simulink model "ControlPendulo2GDL_PL"  (R2019b)
settings: Solver=ode4  StartTime=0.0  StopTime=ts  FixedStep=0.01  RelTol=1e-3
values from neighbouring files (symbols this model uses):
  C = [1 0 0 0]    [PenduloDatos.m]
  K = place(Al,Bl,[Pd1 Pd2 Pd3 Pd4])    [PenduloDatos.m]
  K0 = inv(C*(inv(-Al+Bl*K))*Bl)    [PenduloDatos.m]
  K0D = inv(CD*inv(eye(4)-AD+BD*KD)*BD)    [PenduloDatos.m]
  KD = place(AD,BD,exp([Pd1 Pd2 Pd3 Pd4]*tm))    [PenduloDatos.m]
  L = place(Al',C',[5*Pd1 5*Pd2 5*Pd3 5*Pd4])'    [PenduloDatos.m]
  l1 = c1    (= 0.3)    [PenduloDatos.m]
  l2 = c2    (= 0.2)    [PenduloDatos.m]
  LD = place(AD',CD',exp([5*Pd1 5*Pd2 5*Pd3 5*Pd4]*tm))'    [PenduloDatos.m]
  Ref = 0.2    [PenduloDatos.m]
  tm = 0.01    [PenduloDatos.m]
  XI = [0;0;0;0]    [PenduloDatos.m]
undefined symbols (not defined in the file or in its folder): AD, Al, BD, Bl, CD
libraries: simulink x6
settings Model: Creator=ARQ SEVILLA R  LastModifiedBy=ARQ SEVILLA R

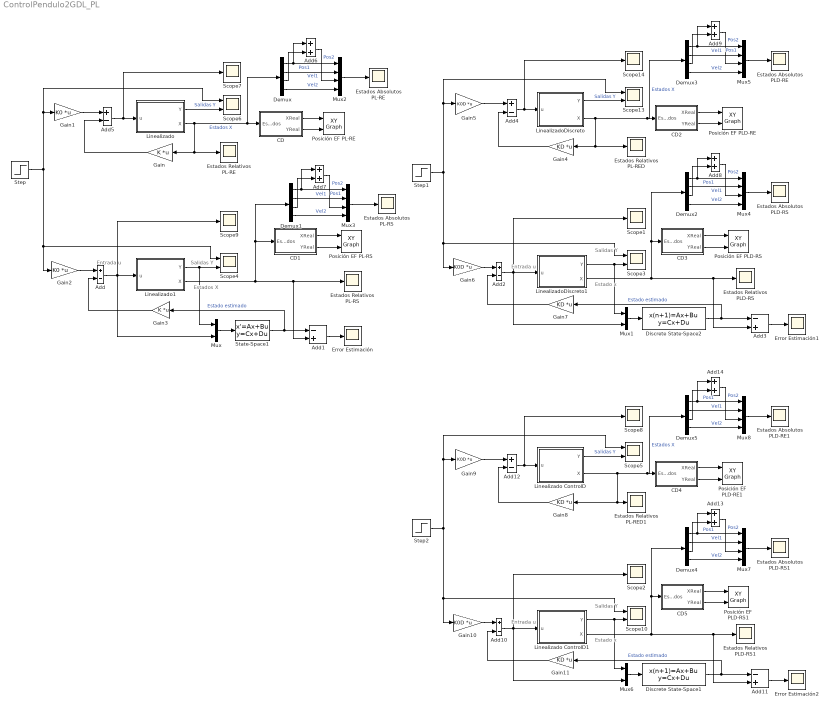
== system ControlPendulo2GDL_PL ==
  note: Estados X
  note: Salidas Y
  note: Entrada u
  note: Salidas Y
  note: Entrada u
  note: Estado x
  note: Entrada u
  note: Estado x
  note: Salidas Y
  Add{,2,4..5,10,12} (6 alike) : Sum  Inputs=+-
  Add1 : Sum  Inputs=-+
  Add11 : Sum  Inputs=-+
  Add{6..9,13..14} (6 alike) : Sum
  Add3 : Sum  Inputs=-+
  CD : Subsystem  TreatAsAtomicUnit=on
  CD1 : Subsystem  TreatAsAtomicUnit=on
  CD2 : Subsystem  TreatAsAtomicUnit=on
  CD3 : Subsystem  TreatAsAtomicUnit=on
  CD4 : Subsystem  TreatAsAtomicUnit=on
  CD5 : Subsystem  TreatAsAtomicUnit=on
  Demux{,1..5} (6 alike) : Demux
  Discrete State-Space1 : DiscreteStateSpace  A=AD-LD*CD  B=[LD BD]  C=eye(4)  D=zeros(4,2)  InitialCondition=XI  SampleTime=tm
  Discrete State-Space2 : DiscreteStateSpace  A=AD-LD*CD  B=[LD BD]  C=eye(4)  D=zeros(4,2)  InitialCondition=XI  SampleTime=tm
  Error Estimación : Scope
  Error Estimación1 : Scope
  Error Estimación2 : Scope
  Estados Absolutos PL-RE : Scope
  Estados Absolutos PL-RS : Scope
  Estados Absolutos PLD-RE : Scope
  Estados Absolutos PLD-RE1 : Scope
  Estados Absolutos PLD-RS : Scope
  Estados Absolutos PLD-RS1 : Scope
  Estados Relativos PL-RE : Scope
  Estados Relativos PL-RED : Scope
  Estados Relativos PL-RED1 : Scope
  Estados Relativos PL-RS : Scope
  Estados Relativos PLD-RS : Scope
  Estados Relativos PLD-RS1 : Scope
  Gain : Gain  Gain=K  Multiplication=Matrix(K*u)
  Gain1 : Gain  Gain=K0  Multiplication=Matrix(K*u)
  Gain{5..6,9..10} (4 alike) : Gain  Gain=K0D  Multiplication=Matrix(K*u)
  Gain{4,7..8,11} (4 alike) : Gain  Gain=KD  Multiplication=Matrix(K*u)
  Gain2 : Gain  Gain=K0  Multiplication=Matrix(K*u)
  Gain3 : Gain  Gain=K  Multiplication=Matrix(K*u)
  Linealizado : Subsystem
  Linealizado ControlD : Subsystem
  Linealizado ControlD1 : Subsystem
  Linealizado1 : Subsystem
  LinealizadoDiscreto : Subsystem
  LinealizadoDiscreto1 : Subsystem
  Mux : Mux  Inputs=2
  Mux1 : Mux  Inputs=2
  Mux{2..5,7..8} (6 alike) : Mux
  Mux6 : Mux  Inputs=2
  Posición EF PL-RE : simulink/Sinks/XY Graph  xmin=-l2-l1  xmax=l2+l1  ymin=-l2-l1  ymax=l2+l1  st=-1
  Posición EF PL-RS : simulink/Sinks/XY Graph  xmin=-l2-l1  xmax=l2+l1  ymin=-l2-l1  ymax=l2+l1  st=-1
  Posición EF PLD-RE : simulink/Sinks/XY Graph  xmin=-l2-l1  xmax=l2+l1  ymin=-l2-l1  ymax=l2+l1  st=-1
  Posición EF PLD-RE1 : simulink/Sinks/XY Graph  xmin=-l2-l1  xmax=l2+l1  ymin=-l2-l1  ymax=l2+l1  st=-1
  Posición EF PLD-RS : simulink/Sinks/XY Graph  xmin=-l2-l1  xmax=l2+l1  ymin=-l2-l1  ymax=l2+l1  st=-1
  Posición EF PLD-RS1 : simulink/Sinks/XY Graph  xmin=-l2-l1  xmax=l2+l1  ymin=-l2-l1  ymax=l2+l1  st=-1
  Scope{1..2,7..9,14} (6 alike) : Scope
  Scope{3..6,10,13} (6 alike) : Scope  NumInputPorts=2
  State-Space1 : StateSpace  A=Al-L*C  B=[L,Bl]  C=eye(4)  D=zeros(4,2)  InitialCondition=XI
  Step : Step  Time=0  After=Ref  SampleTime=0
  Step1 : Step  Time=0  After=Ref  SampleTime=tm
  Step2 : Step  Time=0  After=Ref  SampleTime=tm
  wires:
  Linealizado/2(X) -> Demux/1, CD/1(Estados), Estados Relativos PL-RE/1, Gain/1  "Estados X"
  Add5/1 -> Scope7/1, Linealizado/1(u)
  Gain1/1 -> Add5/1
  Linealizado1/2(X) -> CD1/1(Estados), Demux1/1, Estados Relativos PL-RS/1, Add1/2
  Add/1 -> Scope9/1, Linealizado1/1(u), Mux/2
  Gain2/1 -> Add/1
  Linealizado1/1(Y) -> Mux/1, Scope4/2
  Mux/1 -> State-Space1/1
  Add1/1 -> Error Estimación/1
  Gain3/1 -> Add/2
  State-Space1/1 -> Add1/1, Gain3/1  "Estado estimado"
  CD/1(XReal) -> Posición EF PL-RE/1
  CD/2(YReal) -> Posición EF PL-RE/2
  Step/1 -> Gain2/1, Scope4/1, Scope6/1, Gain1/1
  Linealizado/1(Y) -> Scope6/2  "Salidas Y"
  Gain/1 -> Add5/2
  CD1/2(YReal) -> Posición EF PL-RS/2
  CD1/1(XReal) -> Posición EF PL-RS/1
  LinealizadoDiscreto1/1(Y) -> Mux1/1, Scope3/2
  Gain7/1 -> Add2/2
  LinealizadoDiscreto/1(Y) -> Scope13/2  "Salidas Y"
  Gain6/1 -> Add2/1
  Add2/1 -> Scope1/1, LinealizadoDiscreto1/1(u), Mux1/2
  Add3/1 -> Error Estimación1/1
  Mux1/1 -> Discrete State-Space2/1
  Discrete State-Space2/1 -> Add3/1, Gain7/1  "Estado estimado"
  Gain4/1 -> Add4/2
  Step1/1 -> Scope13/1, Gain5/1, Gain6/1, Scope3/1
  Add4/1 -> LinealizadoDiscreto/1(u), Scope14/1
  Gain5/1 -> Add4/1
  CD2/2(YReal) -> Posición EF PLD-RE/2
  CD2/1(XReal) -> Posición EF PLD-RE/1
  CD3/1(XReal) -> Posición EF PLD-RS/1
  CD3/2(YReal) -> Posición EF PLD-RS/2
  Demux/3 -> Add6/2
  Demux/1 -> Add6/1, Mux2/1  "Pos1"
  Mux2/1 -> Estados Absolutos PL-RE/1
  Demux/2 -> Mux2/2  "Vel1"
  Add6/1 -> Mux2/3  "Pos2"
  Demux/4 -> Mux2/4  "Vel2"
  Demux1/4 -> Mux3/4  "Vel2"
  Add7/1 -> Mux3/3  "Pos2"
  Demux1/2 -> Mux3/2  "Vel1"
  Mux3/1 -> Estados Absolutos PL-RS/1
  Demux1/1 -> Mux3/1, Add7/1  "Pos1"
  Demux1/3 -> Add7/2
  Demux2/3 -> Add8/2
  Demux2/1 -> Add8/1, Mux4/1  "Pos1"
  Mux4/1 -> Estados Absolutos PLD-RS/1
  Demux2/2 -> Mux4/2  "Vel1"
  Add8/1 -> Mux4/3  "Pos2"
  LinealizadoDiscreto1/2(X) -> Estados Relativos PLD-RS/1, Add3/2, Demux2/1, CD3/1(Estados)
  Demux2/4 -> Mux4/4  "Vel2"
  Demux3/4 -> Mux5/4  "Vel2"
  LinealizadoDiscreto/2(X) -> Demux3/1, CD2/1(Estados), Estados Relativos PL-RED/1, Gain4/1  "Estados X"
  Add9/1 -> Mux5/3  "Pos2"
  Demux3/2 -> Mux5/2  "Vel1"
  Mux5/1 -> Estados Absolutos PLD-RE/1
  Demux3/1 -> Mux5/1, Add9/1  "Pos1"
  Demux3/3 -> Add9/2
  Add12/1 -> Linealizado ControlD/1(u), Scope8/1
  Demux4/2 -> Mux7/2  "Vel1"
  Demux4/3 -> Add13/2
  Demux4/1 -> Add13/1, Mux7/1  "Pos1"
  Mux6/1 -> Discrete State-Space1/1
  Linealizado ControlD/1(Y) -> Scope5/2  "Salidas Y"
  Add11/1 -> Error Estimación2/1
  Step2/1 -> Scope5/1, Gain9/1, Gain10/1, Scope10/1
  Add10/1 -> Linealizado ControlD1/1(u), Scope2/1, Mux6/2
  Gain10/1 -> Add10/1
  Linealizado ControlD1/1(Y) -> Mux6/1, Scope10/2
  Demux5/3 -> Add14/2
  Gain9/1 -> Add12/1
  Mux8/1 -> Estados Absolutos PLD-RE1/1
  Linealizado ControlD/2(X) -> Demux5/1, CD4/1(Estados), Gain8/1, Estados Relativos PL-RED1/1  "Estados X"
  Demux5/2 -> Mux8/2  "Vel1"
  Mux7/1 -> Estados Absolutos PLD-RS1/1
  Demux5/1 -> Mux8/1, Add14/1  "Pos1"
  CD4/1(XReal) -> Posición EF PLD-RE1/1
  CD5/2(YReal) -> Posición EF PLD-RS1/2
  Demux4/4 -> Mux7/4  "Vel2"
  CD5/1(XReal) -> Posición EF PLD-RS1/1
  CD4/2(YReal) -> Posición EF PLD-RE1/2
  Gain8/1 -> Add12/2
  Gain11/1 -> Add10/2
  Demux5/4 -> Mux8/4  "Vel2"
  Add14/1 -> Mux8/3  "Pos2"
  Linealizado ControlD1/2(X) -> Estados Relativos PLD-RS1/1, Add11/2, Demux4/1, CD5/1(Estados)
  Discrete State-Space1/1 -> Add11/1, Gain11/1  "Estado estimado"
  Add13/1 -> Mux7/3  "Pos2"

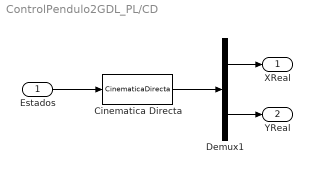
== system ControlPendulo2GDL_PL/CD ==
  Estados : Inport
  Cinematica Directa : MATLABFcn  MATLABFcn=CinematicaDirecta  OutputDimensions=2
  Demux1 : Demux  Outputs=2
  XReal : Outport  VectorParamsAs1DForOutWhenUnconnected=off
  YReal : Outport  Port=2  VectorParamsAs1DForOutWhenUnconnected=off
  wires:
  Cinematica Directa/1 -> Demux1/1
  Demux1/1 -> XReal/1
  Demux1/2 -> YReal/1
  Estados/1 -> Cinematica Directa/1

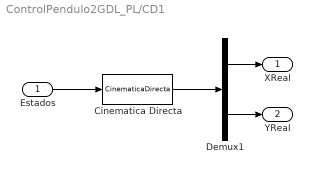
== system ControlPendulo2GDL_PL/CD1 ==
  Estados : Inport
  Cinematica Directa : MATLABFcn  MATLABFcn=CinematicaDirecta  OutputDimensions=2
  Demux1 : Demux  Outputs=2
  XReal : Outport  VectorParamsAs1DForOutWhenUnconnected=off
  YReal : Outport  Port=2  VectorParamsAs1DForOutWhenUnconnected=off
  wires:
  Estados/1 -> Cinematica Directa/1
  Demux1/2 -> YReal/1
  Demux1/1 -> XReal/1
  Cinematica Directa/1 -> Demux1/1

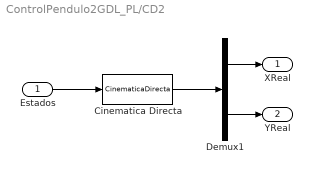
== system ControlPendulo2GDL_PL/CD2 ==
  Estados : Inport
  Cinematica Directa : MATLABFcn  MATLABFcn=CinematicaDirecta  OutputDimensions=2
  Demux1 : Demux  Outputs=2
  XReal : Outport  VectorParamsAs1DForOutWhenUnconnected=off
  YReal : Outport  Port=2  VectorParamsAs1DForOutWhenUnconnected=off
  wires:
  Estados/1 -> Cinematica Directa/1
  Demux1/2 -> YReal/1
  Demux1/1 -> XReal/1
  Cinematica Directa/1 -> Demux1/1

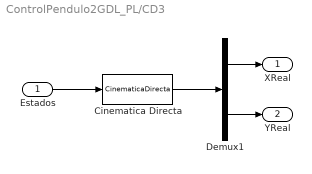
== system ControlPendulo2GDL_PL/CD3 ==
  Estados : Inport
  Cinematica Directa : MATLABFcn  MATLABFcn=CinematicaDirecta  OutputDimensions=2
  Demux1 : Demux  Outputs=2
  XReal : Outport  VectorParamsAs1DForOutWhenUnconnected=off
  YReal : Outport  Port=2  VectorParamsAs1DForOutWhenUnconnected=off
  wires:
  Cinematica Directa/1 -> Demux1/1
  Demux1/1 -> XReal/1
  Demux1/2 -> YReal/1
  Estados/1 -> Cinematica Directa/1

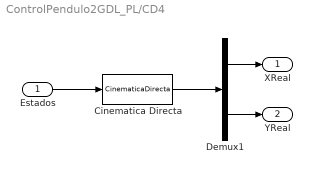
== system ControlPendulo2GDL_PL/CD4 ==
  Estados : Inport
  Cinematica Directa : MATLABFcn  MATLABFcn=CinematicaDirecta  OutputDimensions=2
  Demux1 : Demux  Outputs=2
  XReal : Outport  VectorParamsAs1DForOutWhenUnconnected=off
  YReal : Outport  Port=2  VectorParamsAs1DForOutWhenUnconnected=off
  wires:
  Estados/1 -> Cinematica Directa/1
  Demux1/2 -> YReal/1
  Demux1/1 -> XReal/1
  Cinematica Directa/1 -> Demux1/1

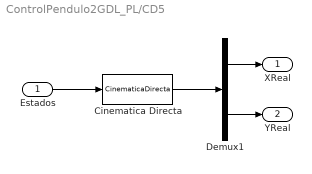
== system ControlPendulo2GDL_PL/CD5 ==
  Estados : Inport
  Cinematica Directa : MATLABFcn  MATLABFcn=CinematicaDirecta  OutputDimensions=2
  Demux1 : Demux  Outputs=2
  XReal : Outport  VectorParamsAs1DForOutWhenUnconnected=off
  YReal : Outport  Port=2  VectorParamsAs1DForOutWhenUnconnected=off
  wires:
  Cinematica Directa/1 -> Demux1/1
  Demux1/1 -> XReal/1
  Demux1/2 -> YReal/1
  Estados/1 -> Cinematica Directa/1

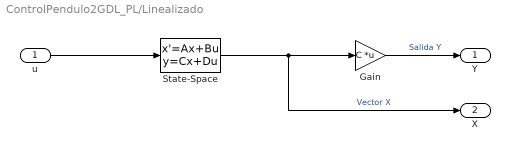
== system ControlPendulo2GDL_PL/Linealizado ==
  u : Inport
  Gain : Gain  Gain=C  Multiplication=Matrix(K*u)
  State-Space : StateSpace  A=Al  B=Bl  C=eye(4)  D=zeros(4,1)  InitialCondition=XI
  Y : Outport
  X : Outport  Port=2
  wires:
  State-Space/1 -> Gain/1, X/1  "Vector X"
  Gain/1 -> Y/1  "Salida Y"
  u/1 -> State-Space/1

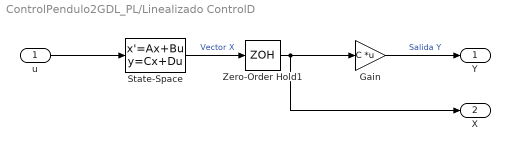
== system ControlPendulo2GDL_PL/Linealizado ControlD ==
  u : Inport
  Gain : Gain  Gain=C  Multiplication=Matrix(K*u)
  State-Space : StateSpace  A=Al  B=Bl  C=eye(4)  D=zeros(4,1)  InitialCondition=XI
  Zero-Order Hold1 : ZeroOrderHold  SampleTime=tm
  Y : Outport
  X : Outport  Port=2
  wires:
  Gain/1 -> Y/1  "Salida Y"
  u/1 -> State-Space/1
  State-Space/1 -> Zero-Order Hold1/1  "Vector X"
  Zero-Order Hold1/1 -> Gain/1, X/1

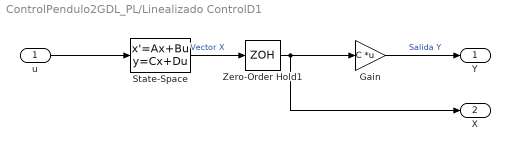
== system ControlPendulo2GDL_PL/Linealizado ControlD1 ==
  u : Inport
  Gain : Gain  Gain=C  Multiplication=Matrix(K*u)
  State-Space : StateSpace  A=Al  B=Bl  C=eye(4)  D=zeros(4,1)  InitialCondition=XI
  Zero-Order Hold1 : ZeroOrderHold  SampleTime=tm
  Y : Outport
  X : Outport  Port=2
  wires:
  Gain/1 -> Y/1  "Salida Y"
  u/1 -> State-Space/1
  State-Space/1 -> Zero-Order Hold1/1  "Vector X"
  Zero-Order Hold1/1 -> Gain/1, X/1

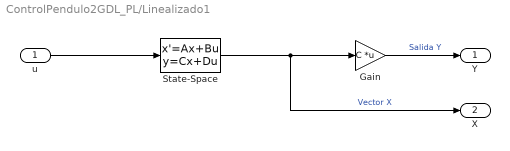
== system ControlPendulo2GDL_PL/Linealizado1 ==
  u : Inport
  Gain : Gain  Gain=C  Multiplication=Matrix(K*u)
  State-Space : StateSpace  A=Al  B=Bl  C=eye(4)  D=zeros(4,1)  InitialCondition=XI
  Y : Outport
  X : Outport  Port=2
  wires:
  u/1 -> State-Space/1
  Gain/1 -> Y/1  "Salida Y"
  State-Space/1 -> Gain/1, X/1  "Vector X"

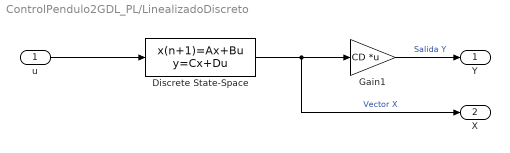
== system ControlPendulo2GDL_PL/LinealizadoDiscreto ==
  u : Inport
  Discrete State-Space : DiscreteStateSpace  A=AD  B=BD  C=eye(4)  D=zeros(4,1)  InitialCondition=XI  SampleTime=tm
  Gain1 : Gain  Gain=CD  Multiplication=Matrix(K*u)
  Y : Outport
  X : Outport  Port=2
  wires:
  Discrete State-Space/1 -> Gain1/1, X/1  "Vector X"
  u/1 -> Discrete State-Space/1
  Gain1/1 -> Y/1  "Salida Y"

== system ControlPendulo2GDL_PL/LinealizadoDiscreto1 ==
  u : Inport
  Discrete State-Space : DiscreteStateSpace  A=AD  B=BD  C=eye(4)  D=zeros(4,1)  InitialCondition=XI  SampleTime=tm
  Gain1 : Gain  Gain=CD  Multiplication=Matrix(K*u)
  Y : Outport
  X : Outport  Port=2
  wires:
  Discrete State-Space/1 -> Gain1/1, X/1  "Vector X"
  Gain1/1 -> Y/1  "Salida Y"
  u/1 -> Discrete State-Space/1
